simulink model "P2001_230205_InstantaneousCostGD1"  (R2022b)
settings: Solver=VariableStepAuto  StartTime=0.0  StopTime=30  RelTol=1e-7
settings Model: Creator=turib  LastModifiedBy=turib
settings HardwareCC: ProdHWDeviceType=AMD->x86-64 (Windows64)

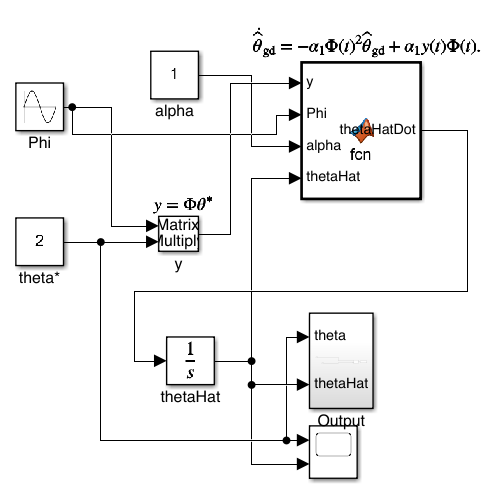
[thumbnail: Simulink's stored preview of the top-level diagram]
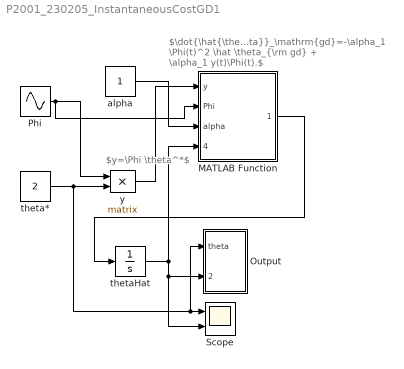
== system P2001_230205_InstantaneousCostGD1 ==
  note: $\dot{\hat{\theta}}_\mathrm{gd}=-\alpha_1 \Phi(t)^2 \hat \theta_{\rm gd} + \alpha_1 y(t)\Phi(t).$
  note: $y=\Phi \theta^*$
  MATLAB Function : MATLAB Function  TreatAsAtomicUnit=on
  Output : Subsystem
  Phi : Sin  Frequency=2  Phase=1  SampleTime=0
  Scope : Scope  NumInputPorts=2
  alpha : Constant
  theta* : Constant  Value=2
  thetaHat : Integrator
  y : Product  Multiplication=Matrix(*)  OutDataTypeStr=double
  wires:
  Phi/1 -> y/1, MATLAB Function/2(Phi)
  theta*/1 -> y/2, Output/1(theta), Scope/1
  MATLAB Function/1(thetaHatDot) -> thetaHat/1
  y/1 -> MATLAB Function/1(y)
  alpha/1 -> MATLAB Function/3(alpha)
  thetaHat/1 -> MATLAB Function/4(thetaHat), Output/2(thetaHat), Scope/2

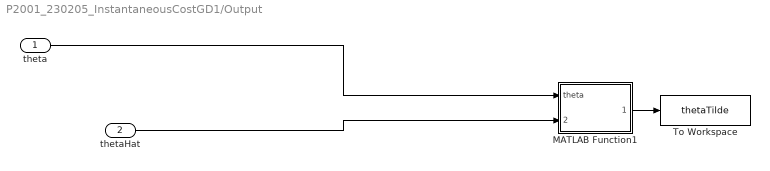
== system P2001_230205_InstantaneousCostGD1/Output ==
  theta : Inport
  thetaHat : Inport  Port=2
  MATLAB Function1 : MATLAB Function  TreatAsAtomicUnit=on
  To Workspace : ToWorkspace  VariableName=thetaTilde  SampleTime=-1
  wires:
  MATLAB Function1/1(thetaTilde) -> To Workspace/1
  thetaHat/1 -> MATLAB Function1/2(thetaHat)
  theta/1 -> MATLAB Function1/1(theta)

== matlab function P2001_230205_InstantaneousCostGD1/MATLAB Function ==
  data: thetaHatDot output; y input; Phi input; alpha input; thetaHat input
function thetaHatDot  = fcn(y, Phi, alpha, thetaHat)
thetaHatDot = - alpha * (Phi ^ 2) * thetaHat + alpha * y * Phi;
end

== matlab function P2001_230205_InstantaneousCostGD1/Output/MATLAB Function1 ==
  data: theta input; thetaTilde output; thetaHat input
function thetaTilde = error(theta, thetaHat)

thetaTilde = thetaHat - theta;

end
